simulink model "polyfit"  (R2022a)
settings: Solver=VariableStepAuto  StartTime=0.0  StopTime=10.0  RelTol=1e-3
libraries: visionsources x1, visionsinks x1
settings Model: Creator=sanz  LastModifiedBy=sanz

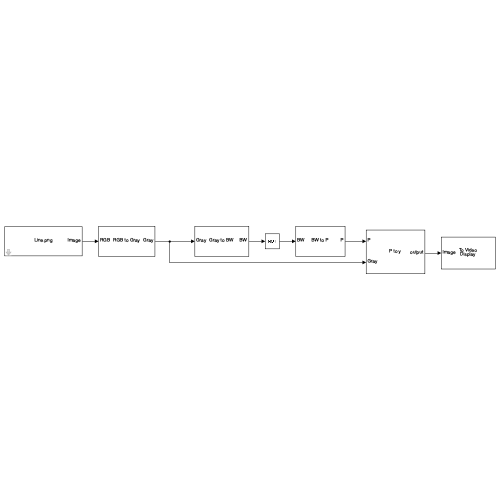
[thumbnail: Simulink's stored preview of the top-level diagram]
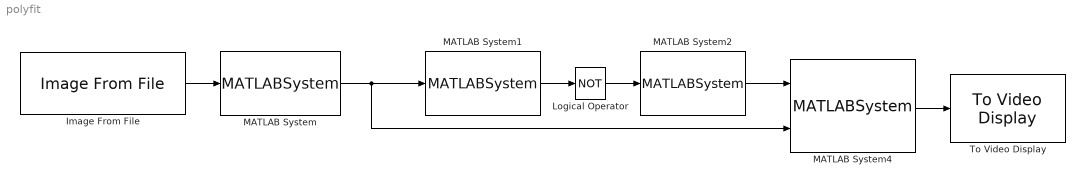
== system polyfit ==
  Image From File : visionsources/Image From File  Tag=vipblks_nd  FileName=/Users/sanz/Desktop/Interface/polyfitmat/Line.png  Ts=10  imagePorts=One multidimensional signal  OutPortLabels=R|G|B  ImageDataType=double  sdImageDataType=uint(8)  Signed=on  WordLength=16  FractionLengthMode=User-defined  FractionLength=15
  Logical Operator : Logic  Operator=NOT  AllPortsSameDT=off  OutDataTypeStr=boolean
  MATLAB System : MATLABSystem  System=Rgb2GraySystem  SimulateUsing=Code generation
      mask Type: Rgb2GraySystem
      mask Display:
      | disp('RGB to Gray');
      | port_label('input',1,'RGB');
      | port_label('output',1,'Gray');
  MATLAB System1 : MATLABSystem  System=FrameBinarizeSystem  SimulateUsing=Code generation
      mask Type: FrameBinarizeSystem
      mask Display:
      | disp('Gray to BW');
      | port_label('input',1,'Gray');
      | port_label('output',1,'BW');
  MATLAB System2 : MATLABSystem  System=PolyfitSystem  Deg=4  SimulateUsing=Code generation
      mask Type: PolyfitSystem
      mask Display:
      | disp('BW to P');
      | port_label('input',1,'BW');
      | port_label('output',1,'P');
  MATLAB System4 : MATLABSystem  System=PolyvalSystem  SimulateUsing=Code generation
      mask Type: PolyvalSystem
      mask Display:
      | disp('P to y');
      | port_label('input',1,'P');
      | port_label('input',2,'Gray');
      | port_label('output',1,'output');
  To Video Display : visionsinks/To Video Display  windowSizeMode=Normal  openAtMdlStart=on  fullScreen=off  videoWindowX=536805376  videoWindowY=536805376  saveWindowSize=off  videoWindowWidth=2147483647  videoWindowHeight=2147483647  inputColorFormat=RGB  inputType=Obsolete  imagePorts=One multidimensional signal  OutputDevice=On-screen video monitor  dataOrg=Column-major  isWindowOpen=off
  wires:
  Image From File/1 -> MATLAB System/1
  MATLAB System4/1 -> To Video Display/1
  MATLAB System1/1 -> Logical Operator/1
  MATLAB System2/1 -> MATLAB System4/1
  Logical Operator/1 -> MATLAB System2/1
  MATLAB System/1 -> MATLAB System1/1, MATLAB System4/2
